simulink model "diff_eq_1"  (R2022a)
settings: Solver=ode45  StartTime=0.0  StopTime=3  RelTol=1e-3
settings Model: Creator=olya-  LastModifiedBy=novik
settings ModelReferenceCC: EnableRefExpFcnMdlSchedulingChecks=off
settings RTWCC: Description=Generic Real-Time Target

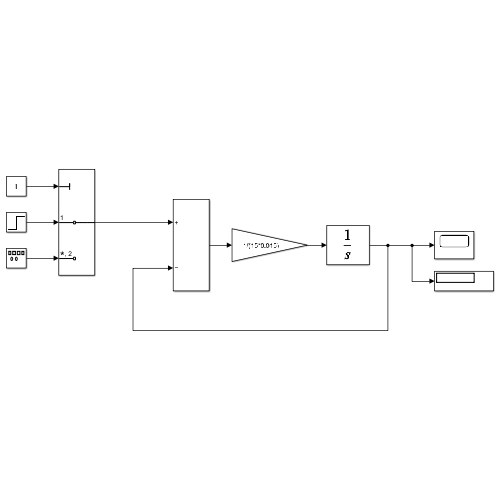
[thumbnail: Simulink's stored preview of the top-level diagram]
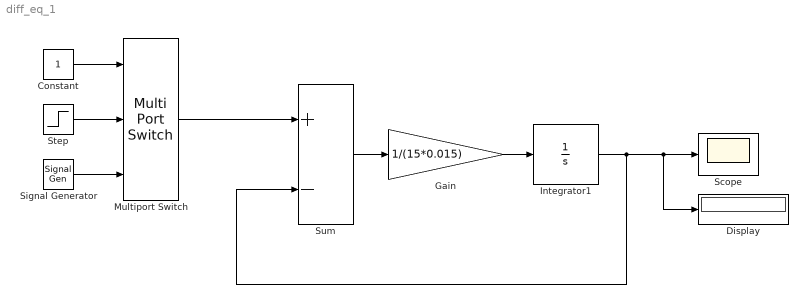
== system diff_eq_1 ==
  Constant : Constant
  Display : Display
      settings: Decimation=50
  Gain : Gain  Gain=1/(15*0.015)  SaturateOnIntegerOverflow=on  OutDataTypeStr=Inherit: Same as input  ParamDataTypeStr=Inherit: Same as input
  Integrator1 : Integrator
  Multiport Switch : MultiPortSwitch  Inputs=2  SaturateOnIntegerOverflow=off  InputSameDT=off
  Scope : Scope
  Signal Generator : SignalGenerator  WaveForm=square  Amplitude=50  Frequency=0.1
  Step : Step  Time=0  After=50  SampleTime=0
  Sum : Sum  Inputs=+-  InputSameDT=on  SaturateOnIntegerOverflow=on  OutDataTypeStr=Inherit: Same as first input
  wires:
  Signal Generator/1 -> Multiport Switch/3
  Step/1 -> Multiport Switch/2
  Constant/1 -> Multiport Switch/1
  Multiport Switch/1 -> Sum/1
  Integrator1/1 -> Sum/2, Display/1, Scope/1
  Sum/1 -> Gain/1
  Gain/1 -> Integrator1/1
